simulink model "main_v8"  (R2022a)
settings: Solver=VariableStepAuto  StartTime=0.0  StopTime=10  MaxStep=1e-3  RelTol=1e-3
model workspace (MATLAB code in the model file):
  | g=9.81;
  | m1=8;
  | L1=0.2;
  | w1=0.04;
  | m2=12;
  | L2=0.6;
  | w2=0.03;
  | theta1_init=0*pi/180;
  | thetaDot1_init=0;
  | theta2_init=0*pi/180;
  | thetaDot2_init=0;
  | theta3_init=70*pi/180;
  | thetaDot3_init=0;
  | % NOW
  | L = [240 800 1050 1175 225 200 235 248]/1000; % m
  | LW = [0 480 0 0 400 100]/1000; % widths
  | M = [150 750 250 150 200 100 0 50]; % mass
  | mM = [0.5 8 8;50 50 50;0.2 1 1;2 3 2; 1 18 18; 0.5 2 2; 0 0 0; 1 1 1;]; % moment mass inertia
  | mMIL3 = [1 20 20; 0.2 1 1;];
  | mML1arm = [10 10 10];
  | ML1arm = 500;
  | CB = 300/1000; % m
  | 
  | % choosen variables
  | JD = 1e5; % join dampening
  | arm_width=0.1;
  | L0 = 750/1000; %m
  | k = 750*1000; %N/m
  | 
  | 
  | P1 = [2000 500 1600];
  | P2 = [2000 -500 1600];
  | P3 = [1600 500 900];
  | P4 = [1600 0 900];
  | P5 = P1;
  | P = [P1; P2; P3; P4; P5;]/1000; % m
undefined symbols (not defined in the file or in its folder): X, Y, Z
libraries: sm_lib x51, nesl_utility x7
(part 2 of 2)

== matlab function main_v8/MATLAB Function ==
  data: x output; t input; y output; z output
function [x,y,z] = fcn(t)
a_x = [2; -1.38777878078145e-17; 0; 0.0199999999999998; -0.00999999999999992];
b_x = [1.44000000000001; 0.759999999999989; -0.299999999999995; 0.0299999999999993];
c_x = [2.07999999999982; 0.280000000000129; -0.180000000000030; 0.0200000000000023];
d_x = [99.2800000000026; -56.9600000000014; 12.2400000000003; -1.15000000000003; 0.0400000000000009];

a_y = [0.500000000000000; 0; 0; -0.412500000000000; 0.143750000000000];
b_y = [6.300000000000017; -7.550000000000020; 2.625000000000008; -0.275000000000001];
c_y = [-24.900000000000270; 15.850000000000199; -3.225000000000047; 0.212500000000004];
d_y = [2.181000000000052e+02;-1.232000000000029e+02;25.800000000000590;-2.375000000000054;0.081250000000002];

a_z = [1.600000000000000; 0; 0; 0.035000000000000; -0.017500000000000];
b_z = [0.620000000000010; 1.329999999999986; -0.524999999999994; 0.052499999999999];
c_z = [1.739999999999777; 0.490000000000161; -0.315000000000038; 0.035000000000003];
d_z = [1.718400000000044e+02; -99.680000000002420; 21.420000000000503; -2.012500000000046; 0.070000000000002];
x=2;
y=0.5;
z=1.6;
if t <= 2
    x = F4(t)*a_x;
    y = F4(t)*a_y;
    z = F4(t)*a_z;
elseif t <= 4
    x = F3(t)*b_x;
    y = F3(t)*b_y;
    z = F3(t)*b_z;
elseif t <= 6
    x = F3(t)*c_x;
    y = F3(t)*c_y;
    z = F3(t)*c_z;
elseif t <= 8
    x = F4(t)*d_x;
    y = F4(t)*d_y;
    z = F4(t)*d_z;
end
end

function [out] = F4(t) 
out = [1 t t.^2 t.^3 t.^4];
end

function [out] = F3(t) 
out = [1 t t.^2 t.^3];
end
